simulink model "mpu6050_working_copy"  (R2017a)
settings: Solver=FixedStepDiscrete  StartTime=0.0  StopTime=inf  RelTol=1e-3
PostLoadFcn:
  | ChipSelect = 1;  % choose I2C comms
  | AddressAlt = 0;  % use default address
  | 
  | if AddressAlt == 1
  | % b1101001 (pin AD0 is logic high).
  | SlvAddr = uint8(bin2dec('1101001'));  % ADDR ALT = 1
  | else
  | % b1101000 (pin AD0 is logic low)
  | SlvAddr = uint8(bin2dec('1101000'));  % ADDR ALT = 0
  | end
  | SlvAddr = uint8(hex2dec('68'));
  | 
  | 
  | % 0x3B 59 ACCEL_XOUT[15:8]
  | % 0x3C 60 ACCEL_XOUT[7:0]
  | % 0x3D 61 ACCEL_YOUT[15:8]
  | % 0x3E 62 ACCEL_YOUT[7:0]
  | % 0x3F 63 ACCEL_ZOUT[15:8]
  | % 0x40 64 ACCEL_ZOUT[7:0]
  | 
  | AccelXRegAddr = uint8(hex2dec('3B'));
  | AccelYRegAddr = uint8(hex2dec('3D'));
  | AccelZRegAddr = uint8(hex2dec('3F'));
  | 
  | % 0x43 67 GYRO_XOUT[15:8]
  | % 0x44 68 GYRO_XOUT[7:0]
  | % 0x45 69 GYRO_YOUT[15:8]
  | % 0x46 70 GYRO_YOUT[7:0]
  | % 0x47 71 GYRO_ZOUT[15:8]
  | % 0x48 72 GYRO_ZOUT[7:0]
  | 
  | GyroXRegAddr = uint8(hex2dec('43'));
  | GyroYRegAddr = uint8(hex2dec('45'));
  | GyroZRegAddr = uint8(hex2dec('47'));
  | 
  | deviceAddr = fi(SlvAddr,0,7,0);
  | 
  | powerRegAddr = uint8(hex2dec('6B'));
  | powerRegData = bin2dec('10000001');
(part 2 of 2)

== stateflow chart mpu6050_working_copy/I2C_MPU6050_IP/MPU6050_Interface1 ==
  settings: executeAtInitialization=1
  state init
    %initstate
    Valid_Out = 0;
    selfInit = 1;
    slv_addr = SlvAddr;
    %TODO delete all
    tmp = 0;
    tmpConfig = 0;
    tmpReadGyro = 0;
    tmpReadAccel = 0;
    tmpValid = 0;
    tmpReadDevice = 0;
    tmpHere = 0;
  note: I2C Configuration for MPU6050
  note: 0x3B 59 ACCEL_XOUT[15:8]
      | 0x3C 60 ACCEL_XOUT[7:0]
      | 0x3D 61 ACCEL_YOUT[15:8]
      | 0x3E 62 ACCEL_YOUT[7:0]
      | 0x3F 63 ACCEL_ZOUT[15:8]
      | 0x40 64 ACCEL_ZOUT[7:0]
      |
      | 0x43 67 GYRO_XOUT[15:8]
      | 0x44 68 GYRO_XOUT[7:0]
      | 0x45 69 GYRO_YOUT[15:8]
      | 0x46 70 GYRO_YOUT[7:0]
      | 0x47 71 GYRO_ZOUT[15:8]
      | 0x48 72 GYRO_ZOUT[7:0]
      |
      | 0x6B 107 PWR_MGMT_1
      | 0x6C 108 PWR_MGMT_2
  state idle
    %idlestate
    enb 	= 0;
    rw 		= 0;
    mode 	= 0;
    cnt      = 0;
    reg_byte_mode = 0;
  state ReadDeviceData [group]
    note: DEVID is an example of
        | doing a 1-byte READ
    note: 0x75 117 - WHO_AM_I[6:1]
    state getDEVID
      entry:
      enb = 1;
      rw = 1;
      mode = 0;
      reg_addr =   uint8(117);
      tmpReadDevice = 1;
    state waitforNotBusy1
      enb=0;
    state readDEVID
      deviceId = uint8(data_in);
      tmpHere = 1;
    state waitforNotBusy6
      enb=0;
    state getRegData
      entry:
      enb = 1;
      rw = 1;
      mode = 0;
      reg_addr = userRegAddr;
    state waitforNotBusy5
      enb=0;
    state readUserRegData
      regdata = uint8(data_in);
    getDEVID -> waitforNotBusy1 : [busy==1]
    waitforNotBusy1 -> readDEVID [order 1] : [mstr_ack==1]
    waitforNotBusy1 -> waitforNotBusy6 [order 2] : [n_ack==1]
    readDEVID -> getRegData : [busy==0]
    waitforNotBusy6 -> (junction 2281) : [busy==0 || busy == 1]
    getRegData -> waitforNotBusy5 : [busy==1]
    waitforNotBusy5 -> readUserRegData [order 1] : [mstr_ack==1]
    waitforNotBusy5 -> (junction 2281) [order 2] : [n_ack==1]
  state Configuration [group]
    state setPwrMode
      enb = 1;
      rw = 0;
      mode = 0;
      reg_addr = powerRegAddr;
      data_out = powerRegData;
      tmpConfig = 1;
    state waitforNotBusy2
      enb=0;
    state setDataFormat [commented out]
      enb = 1;
      rw = 0;
      mode = 0;
      reg_addr = uint8(49); % 0x31
      data_out = uint8(0); % or 0x08
    state waitforNotBusy3 [commented out]
      enb=0;
    state setFIFOCfg [commented out]
      enb = 1;
      rw = 0;
      mode = 0;
      reg_addr = uint8(56); % 0x38
      data_out = uint8(8); % 0x08
    state waitforNotBusy4 [commented out]
      enb=0;
    state cfgDone
      selfInit = 0;
      tmp = 1;
    setPwrMode -> Configuration.waitforNotBusy2 : [busy==1]
    Configuration.waitforNotBusy2 -> (junction 2329) [order 2] : [busy==0]
    Configuration.waitforNotBusy2 -> (junction 2279) [order 1] : [n_ack==1]
    waitforNotBusy3 -> (junction 2279) [commented out] : [n_ack==1]
    waitforNotBusy4 -> (junction 2279) [commented out] : [n_ack==1]
    setDataFormat -> waitforNotBusy3 [commented out] : [busy==1]
    waitforNotBusy3 -> setFIFOCfg [commented out] : [busy==0]
    (junction 2329) -> Configuration.cfgDone
    setFIFOCfg -> waitforNotBusy4 [commented out] : [busy==1]
  state cfgDone
    selfInit = 0;
    tmp = 1;
  state check_cfg
    en: enb = 0;
    cnt = 0;
    du: cnt = cnt + 1;
    tmpCheckCng = 1
  state ReadAccelData [group]
    state read_accelX_registers0
      entry:
      enb = 1;
      rw = 1;
      mode = 1;
      reg_addr =  AccelXRegAddr;
      Valid_Out = 0;
      tmpReadAccel = 1;
    state waitforNotBusy2
      enb=0;
    state accelX_LSB
      tempVal = data_in;
    state toggle
    state accelX_MSB
      AccelX =  convert_int16(tempVal, data_in);
    state toggle3
    state accelY_LSB
      tempVal = data_in;
    state toggle1
    state accelY_MSB
      AccelY = convert_int16(tempVal,data_in);
    state toggle4
    state accelZ_LSB
      tempVal = data_in;
    state toggle2
      mode = 0;
    state accelZ_MSB
      AccelZ =  convert_int16(tempVal, data_in);
    read_accelX_registers0 -> ReadAccelData.waitforNotBusy2 : [busy==1]
    ReadAccelData.waitforNotBusy2 -> accelX_LSB [order 1] : [mstr_ack==1]
    accelX_LSB -> ReadAccelData.toggle : [mstr_ack==0]
    ReadAccelData.toggle -> accelX_MSB : [mstr_ack==1]
    accelX_MSB -> ReadAccelData.toggle3 [order 2] : [mstr_ack==0]
    accelX_MSB -> (junction 2286) [order 1] : [n_ack==1]
    ReadAccelData.toggle3 -> accelY_LSB : [mstr_ack==1]
    accelY_LSB -> ReadAccelData.toggle1 : [mstr_ack==0]
    ReadAccelData.toggle1 -> accelY_MSB : [mstr_ack==1]
    accelY_MSB -> (junction 2286) [order 1] : [n_ack==1]
    accelZ_MSB -> (junction 2286) [order 1] : [n_ack==1]
    accelY_MSB -> ReadAccelData.toggle4 [order 2] : [mstr_ack==0]
    ReadAccelData.toggle4 -> accelZ_LSB : [mstr_ack==1]
    accelZ_LSB -> ReadAccelData.toggle2 : [mstr_ack==0]
    ReadAccelData.toggle2 -> accelZ_MSB : [mstr_ack==1]
  state Valid
    en: enb = 0;
    cnt = 0;
    Valid_Out = 1;
    du: cnt = cnt + 1;
    tmpValid = 1;
  state ReadGyroData [group]
    state read_gyroX_registers0
      entry:
      enb = 1;
      rw = 1;
      mode = 1;
      reg_addr =  GyroXRegAddr;
      Valid_Out = 0;
      tmpReadGyro = 1;
    state waitforNotBusy2
      enb=0;
    state gyroX_LSB
      tempVal = data_in;
    state toggle
    state gyroX_MSB
      GyroX =  convert_int16(tempVal, data_in);
    state toggle3
    state gyroY_LSB
      tempVal = data_in;
    state toggle1
    state gyroY_MSB
      GyroY = convert_int16(tempVal, data_in);
    state toggle4
    state gyroZ_LSB
      tempVal = data_in;
    state toggle2
      mode = 0;
    state gyroZ_MSB
      GyroZ =  convert_int16(tempVal, data_in);
    read_gyroX_registers0 -> ReadGyroData.waitforNotBusy2 : [busy==1]
    ReadGyroData.waitforNotBusy2 -> gyroX_LSB : [mstr_ack==1]
    gyroX_LSB -> ReadGyroData.toggle : [mstr_ack==0]
    ReadGyroData.toggle -> gyroX_MSB : [mstr_ack==1]
    gyroX_MSB -> ReadGyroData.toggle3 [order 2] : [mstr_ack==0]
    gyroX_MSB -> (junction 2301) [order 1] : [n_ack==1]
    ReadGyroData.toggle3 -> gyroY_LSB : [mstr_ack==1]
    gyroY_LSB -> ReadGyroData.toggle1 : [mstr_ack==0]
    ReadGyroData.toggle1 -> gyroY_MSB : [mstr_ack==1]
    gyroY_MSB -> (junction 2301) [order 1] : [n_ack==1]
    gyroZ_MSB -> (junction 2301) [order 1] : [n_ack==1]
    gyroY_MSB -> ReadGyroData.toggle4 [order 2] : [mstr_ack==0]
    ReadGyroData.toggle4 -> gyroZ_LSB : [mstr_ack==1]
    gyroZ_LSB -> ReadGyroData.toggle2 : [mstr_ack==0]
    ReadGyroData.toggle2 -> gyroZ_MSB : [mstr_ack==1]
  (default) -> init
  init -> idle
  check_cfg -> idle : [cnt >=5]
  idle -> setPwrMode [order 1] : [busy==0 & (configDevice==1 | selfInit == 1)]
  idle -> getDEVID [order 2] : [busy==0]
  readUserRegData -> read_accelX_registers0 : [busy==0]
  (junction 2281) -> check_cfg
  (junction 2286) -> check_cfg
  (junction 2279) -> check_cfg
  ReadAccelData.waitforNotBusy2 -> check_cfg [order 2] : [n_ack==1]
  Valid -> check_cfg : [cnt >= 5]
  Configuration.cfgDone -> read_accelX_registers0
  accelZ_MSB -> read_gyroX_registers0 [order 2] : [busy==0]
  gyroZ_MSB -> Valid [order 2]
  data: msb function_input uint8; lsb function_input uint8; val function_output int16; enb output boolean size=1; rw output boolean size=1; mode output boolean size=1; slv_addr output uint8; reg_addr output uint8; reg_byte_mode output boolean size=1; data_out output uint8; busy input; n_ack input; byte_mode input boolean size=1; reg_mode input boolean size=1; cnt local uint32; data_in input uint8 size=1; mstr_ack input; AccelX output int16; AccelY output int16; AccelZ output int16; SlvAddr parameter uint8; AccelXRegAddr parameter uint8; AccelYRegAddr parameter uint8; AccelZRegAddr parameter uint8; Valid_Out output boolean; tempVal local uint8; deviceId output uint8; powerRegData parameter uint8; regdata output uint8; userRegAddr input uint8; powerRegAddr parameter uint8; configDevice input boolean; selfInit local boolean; GyroXRegAddr parameter uint8; GyroX output int16; GyroY output int16; GyroZ output int16; tmp output boolean; tmpConfig output boolean; tmpCheckCng output boolean; tmpReadGyro output boolean; tmpReadAccel output boolean; tmpValid output boolean; tmpReadDevice output boolean; tmpHere output boolean
  function val = convert_int16(msb, lsb):
    | function val = convert_int16(msb, lsb)
    | 
    | val = int16(bitor(bitshift(int16(msb),8), int16(lsb)));

== stateflow chart mpu6050_working_copy/I2C_MPU6050_IP/MPU6050_Interface2 ==
  settings: executeAtInitialization=1
  state init
    %initstate
    Valid_Out = 0;
    selfInit = 1;
    slv_addr = SlvAddr;
    %TODO delete all
    tmp = 0;
    tmpConfig = 0;
    tmpReadGyro = 0;
    tmpReadAccel = 0;
    tmpValid = 0;
    tmpReadDevice = 0;
    tmpHere = 0;
  state idle1 [commented out]
    %idlestate
    enb 	= 0;
    rw 		= 0;
    mode 	= 0;
    cnt      = 0;
    reg_byte_mode = 0;
  state WriteByteExample [group] [commented out]
    state exPowerMOde [commented out]
      enb = 1;
      rw = 0;
      mode = 0;
      reg_addr = hex2dec('6B');
      data_out = hex2dec('80');
    state waitforNotBusy2 [commented out]
      enb=0;
    state waitforNotBusy3 [commented out]
      enb=0;
    exPowerMOde -> WriteByteExample.waitforNotBusy2 [commented out] : [busy==1]
    WriteByteExample.waitforNotBusy2 -> WriteByteExample.waitforNotBusy3 [commented out] : [busy==0]
  note: I2C Configuration for MPU6050
  note: 0x3B 59 ACCEL_XOUT[15:8]
      | 0x3C 60 ACCEL_XOUT[7:0]
      | 0x3D 61 ACCEL_YOUT[15:8]
      | 0x3E 62 ACCEL_YOUT[7:0]
      | 0x3F 63 ACCEL_ZOUT[15:8]
      | 0x40 64 ACCEL_ZOUT[7:0]
      |
      | 0x43 67 GYRO_XOUT[15:8]
      | 0x44 68 GYRO_XOUT[7:0]
      | 0x45 69 GYRO_YOUT[15:8]
      | 0x46 70 GYRO_YOUT[7:0]
      | 0x47 71 GYRO_ZOUT[15:8]
      | 0x48 72 GYRO_ZOUT[7:0]
      |
      | 0x6B 107 PWR_MGMT_1
      | 0x6C 108 PWR_MGMT_2
  state idle
    %idlestate
    enb 	= 0;
    rw 		= 0;
    mode 	= 0;
    cnt      = 0;
    reg_byte_mode = 0;
  state ReadDeviceData [group]
    note: DEVID is an example of
        | doing a 1-byte READ
    note: 0x75 117 - WHO_AM_I[6:1]
    state getDEVID
      entry:
      enb = 1;
      rw = 1;
      mode = 0;
      reg_addr =   uint8(117);
      tmpReadDevice = 1;
    state waitforNotBusy1
      enb=0;
    state readDEVID
      deviceId = uint8(data_in);
      tmpHere = 1;
    state waitforNotBusy6
      enb=0;
    state getRegData
      entry:
      enb = 1;
      rw = 1;
      mode = 0;
      reg_addr = userRegAddr;
    state waitforNotBusy5
      enb=0;
    state readUserRegData
      regdata = uint8(data_in);
    getDEVID -> waitforNotBusy1 : [busy==1]
    waitforNotBusy1 -> readDEVID [order 1] : [mstr_ack==1]
    waitforNotBusy1 -> ReadDeviceData.waitforNotBusy6 [order 2] : [n_ack==1]
    readDEVID -> getRegData : [busy==0]
    ReadDeviceData.waitforNotBusy6 -> (junction 2281) : [busy==0 || busy == 1]
    getRegData -> ReadDeviceData.waitforNotBusy5 : [busy==1]
    ReadDeviceData.waitforNotBusy5 -> readUserRegData [order 1] : [mstr_ack==1]
    ReadDeviceData.waitforNotBusy5 -> (junction 2281) [order 2] : [n_ack==1]
  state Configuration [group]
    state setPwrMode
      enb = 1;
      rw = 0;
      mode = 0;
      reg_addr = powerRegAddr;
      data_out = powerRegData;
      tmpConfig = 1;
    state waitforNotBusy2
      enb=0;
    state setDataFormat [commented out]
      enb = 1;
      rw = 0;
      mode = 0;
      reg_addr = uint8(49); % 0x31
      data_out = uint8(0); % or 0x08
    state waitforNotBusy3 [commented out]
      enb=0;
    state setFIFOCfg [commented out]
      enb = 1;
      rw = 0;
      mode = 0;
      reg_addr = uint8(56); % 0x38
      data_out = uint8(8); % 0x08
    state waitforNotBusy4 [commented out]
      enb=0;
    state cfgDone
      selfInit = 0;
      tmp = 1;
    setPwrMode -> Configuration.waitforNotBusy2 : [busy==1]
    Configuration.waitforNotBusy2 -> (junction 2329) [order 2] : [busy==0]
    Configuration.waitforNotBusy2 -> (junction 2279) [order 1] : [n_ack==1]
    Configuration.waitforNotBusy3 -> (junction 2279) [commented out] : [n_ack==1]
    Configuration.waitforNotBusy4 -> (junction 2279) [commented out] : [n_ack==1]
    setDataFormat -> Configuration.waitforNotBusy3 [commented out] : [busy==1]
    Configuration.waitforNotBusy3 -> setFIFOCfg [commented out] : [busy==0]
    (junction 2329) -> cfgDone
    setFIFOCfg -> Configuration.waitforNotBusy4 [commented out] : [busy==1]
  state check_cfg
    en: enb = 0;
    cnt = 0;
    du: cnt = cnt + 1;
    tmpCheckCng = 1
  state ReadAccelData [group]
    state read_accelX_registers0
      entry:
      enb = 1;
      rw = 1;
      mode = 1;
      reg_addr =  AccelXRegAddr;
      Valid_Out = 0;
      tmpReadAccel = 1;
    state waitforNotBusy2
      enb=0;
    state accelX_LSB
      tempVal = data_in;
    state toggle
    state accelX_MSB
      AccelX =  convert_int16(tempVal, data_in);
    state toggle3
    state accelY_LSB
      tempVal = data_in;
    state toggle1
    state accelY_MSB
      AccelY = convert_int16(tempVal,data_in);
    state toggle4
    state accelZ_LSB
      tempVal = data_in;
    state toggle2
      mode = 0;
    state accelZ_MSB
      AccelZ =  convert_int16(tempVal, data_in);
    read_accelX_registers0 -> ReadAccelData.waitforNotBusy2 : [busy==1]
    ReadAccelData.waitforNotBusy2 -> accelX_LSB [order 1] : [mstr_ack==1]
    accelX_LSB -> ReadAccelData.toggle : [mstr_ack==0]
    ReadAccelData.toggle -> accelX_MSB : [mstr_ack==1]
    accelX_MSB -> ReadAccelData.toggle3 [order 2] : [mstr_ack==0]
    accelX_MSB -> (junction 2286) [order 1] : [n_ack==1]
    ReadAccelData.toggle3 -> accelY_LSB : [mstr_ack==1]
    accelY_LSB -> ReadAccelData.toggle1 : [mstr_ack==0]
    ReadAccelData.toggle1 -> accelY_MSB : [mstr_ack==1]
    accelY_MSB -> (junction 2286) [order 1] : [n_ack==1]
    accelZ_MSB -> (junction 2286) [order 1] : [n_ack==1]
    accelY_MSB -> ReadAccelData.toggle4 [order 2] : [mstr_ack==0]
    ReadAccelData.toggle4 -> accelZ_LSB : [mstr_ack==1]
    accelZ_LSB -> ReadAccelData.toggle2 : [mstr_ack==0]
    ReadAccelData.toggle2 -> accelZ_MSB : [mstr_ack==1]
  state WriteByteExample [group] [commented out]
    state waitforNotBusy4 [commented out]
      enb=0;
    state resetPowerMode [commented out]
      enb = 1;
      rw = 0;
      mode = 0;
      reg_addr = 107; %0x6B
      data_out = 128; %0x80
    state setClockSource1 [commented out]
      enb = 1;
      rw = 0;
      mode = 0;
      reg_addr = 107; %0x6B
      data_out = 1; %0x01
    state waitforNotBusy5 [commented out]
      enb=0;
    state setClockSource2Maybe [commented out]
      enb = 1;
      rw = 0;
      mode = 0;
      reg_addr = 108; %0x6C
      data_out = 0; %0x00
    state waitforNotBusy6 [commented out]
      enb=0;
    state clearSleepEnableSensors [commented out]
      enb = 1;
      rw = 0;
      mode = 0;
      reg_addr = 107; %0x6B
      data_out = 0; %0x0
    state waitforNotBusy6B [commented out]
      enb=0;
    state configGyroAndAccel1 [commented out]
      enb = 1;
      rw = 0;
      mode = 0;
      reg_addr = 107; %0x6B
      data_out = 1; %0x01
    state waitforNotBusy7 [commented out]
      enb=0;
    state configGyroAndAccel [commented out]
      enb = 1;
      rw = 0;
      mode = 0;
      reg_addr = 26; %0x1A
      data_out = 3; %0x03
    state waitforNotBusy8 [commented out]
      enb=0;
    state setSampleRate [commented out]
      %200hz
      enb = 1;
      rw = 0;
      mode = 0;
      reg_addr = 25; %0x19
      data_out = 4; %0x04
    state waitforNotBusy9 [commented out]
      enb=0;
    state setupInterrupts [commented out]
      enb = 1;
      rw = 0;
      mode = 0;
      reg_addr = 55; %0x37
      data_out = 2; %0x02
    state waitforNotBusy10 [commented out]
      enb=0;
    state enableInterrupts [commented out]
      enb = 1;
      rw = 0;
      mode = 0;
      reg_addr = 56; %0x38
      data_out = 1; %0x01
    WriteByteExample.waitforNotBusy4 -> WriteByteExample.setClockSource1 [commented out] : [busy==0]
    WriteByteExample.resetPowerMode -> WriteByteExample.waitforNotBusy4 [commented out] : [busy==1]
    WriteByteExample.setClockSource1 -> WriteByteExample.waitforNotBusy5 [commented out] : [busy==1]
    WriteByteExample.waitforNotBusy5 -> WriteByteExample.setClockSource2Maybe [commented out] : [busy==0]
    WriteByteExample.waitforNotBusy6 -> WriteByteExample.clearSleepEnableSensors [commented out] : [busy==0]
    WriteByteExample.setClockSource2Maybe -> WriteByteExample.waitforNotBusy6 [commented out] : [busy==1]
    WriteByteExample.clearSleepEnableSensors -> WriteByteExample.waitforNotBusy6B [commented out] : [busy==1]
    WriteByteExample.waitforNotBusy6B -> WriteByteExample.configGyroAndAccel1 [commented out] : [busy==0]
    WriteByteExample.waitforNotBusy7 -> configGyroAndAccel [commented out] : [busy==0]
    WriteByteExample.configGyroAndAccel1 -> WriteByteExample.waitforNotBusy7 [commented out] : [busy==1]
    waitforNotBusy8 -> setSampleRate [commented out] : [busy==0]
    configGyroAndAccel -> waitforNotBusy8 [commented out] : [busy==1]
    setSampleRate -> waitforNotBusy9 [commented out] : [busy==1]
    waitforNotBusy9 -> setupInterrupts [commented out] : [busy==0]
    waitforNotBusy10 -> enableInterrupts [commented out] : [busy==0]
    setupInterrupts -> waitforNotBusy10 [commented out] : [busy==1]
  state WriteByteExample [group]
    state waitforNotBusy4
      enb=0;
    state resetPowerMode
      enb = 1;
      rw = 0;
      mode = 0;
      reg_addr = 107; %0x6B
      data_out = 128; %0x80
    state setClockSource1
      enb = 1;
      rw = 0;
      mode = 0;
      reg_addr = 107; %0x6B
      data_out = 1; %0x01
    state waitforNotBusy5
      enb=0;
    state setClockSource2Maybe
      enb = 1;
      rw = 0;
      mode = 0;
      reg_addr = 108; %0x6C
      data_out = 0; %0x00
    state waitforNotBusy6
      enb=0;
    state clearSleepEnableSensors
      enb = 1;
      rw = 0;
      mode = 0;
      reg_addr = 27; %0x6B
      data_out = 0; %0x0
    state waitforNotBusy6B
      enb=0;
    state configGyroAndAccel1
      enb = 1;
      rw = 0;
      mode = 0;
      reg_addr = 28; %0x6B
      data_out = 0; %0x01
    state waitforNotBusy7
      enb=0;
    WriteByteExample.waitforNotBusy4 -> WriteByteExample.setClockSource1 : [busy==0]
    WriteByteExample.resetPowerMode -> WriteByteExample.waitforNotBusy4 : [busy==1]
    WriteByteExample.setClockSource1 -> WriteByteExample.waitforNotBusy5 : [busy==1]
    WriteByteExample.waitforNotBusy5 -> WriteByteExample.setClockSource2Maybe : [busy==0]
    WriteByteExample.waitforNotBusy6 -> WriteByteExample.clearSleepEnableSensors : [busy==0]
    WriteByteExample.setClockSource2Maybe -> WriteByteExample.waitforNotBusy6 : [busy==1]
    WriteByteExample.clearSleepEnableSensors -> WriteByteExample.waitforNotBusy6B : [busy==1]
    WriteByteExample.waitforNotBusy6B -> WriteByteExample.configGyroAndAccel1 : [busy==0]
    WriteByteExample.configGyroAndAccel1 -> WriteByteExample.waitforNotBusy7 : [busy==1]
  state Valid
    en: enb = 0;
    cnt = 0;
    Valid_Out = 1;
    du: cnt = cnt + 1;
    tmpValid = 1;
  state ReadGyroData [group]
    state read_gyroX_registers0
      entry:
      enb = 1;
      rw = 1;
      mode = 1;
      reg_addr =  GyroXRegAddr;
      Valid_Out = 0;
      tmpReadGyro = 1;
    state waitforNotBusy2
      enb=0;
    state gyroX_LSB
      tempVal = data_in;
    state toggle
    state gyroX_MSB
      GyroX =  convert_int16(tempVal, data_in);
    state toggle3
    state gyroY_LSB
      tempVal = data_in;
    state toggle1
    state gyroY_MSB
      GyroY = convert_int16(tempVal, data_in);
    state toggle4
    state gyroZ_LSB
      tempVal = data_in;
    state toggle2
      mode = 0;
    state gyroZ_MSB
      GyroZ =  convert_int16(tempVal, data_in);
    read_gyroX_registers0 -> ReadGyroData.waitforNotBusy2 : [busy==1]
    ReadGyroData.waitforNotBusy2 -> gyroX_LSB : [mstr_ack==1]
    gyroX_LSB -> ReadGyroData.toggle : [mstr_ack==0]
    ReadGyroData.toggle -> gyroX_MSB : [mstr_ack==1]
    gyroX_MSB -> ReadGyroData.toggle3 [order 2] : [mstr_ack==0]
    gyroX_MSB -> (junction 2301) [order 1] : [n_ack==1]
    ReadGyroData.toggle3 -> gyroY_LSB : [mstr_ack==1]
    gyroY_LSB -> ReadGyroData.toggle1 : [mstr_ack==0]
    ReadGyroData.toggle1 -> gyroY_MSB : [mstr_ack==1]
    gyroY_MSB -> (junction 2301) [order 1] : [n_ack==1]
    gyroZ_MSB -> (junction 2301) [order 1] : [n_ack==1]
    gyroY_MSB -> ReadGyroData.toggle4 [order 2] : [mstr_ack==0]
    ReadGyroData.toggle4 -> gyroZ_LSB : [mstr_ack==1]
    gyroZ_LSB -> ReadGyroData.toggle2 : [mstr_ack==0]
    ReadGyroData.toggle2 -> gyroZ_MSB : [mstr_ack==1]
  (default) -> init
  idle1 -> exPowerMOde [commented out]
  init -> idle
  check_cfg -> idle : [cnt >=5]
  idle -> setPwrMode [order 1] : [busy==0 && (configDevice==1 || selfInit == 1)]
  idle -> getDEVID [order 2] : [busy==0]
  readUserRegData -> read_accelX_registers0 : [busy==0]
  (junction 2281) -> check_cfg
  (junction 2286) -> check_cfg
  (junction 2279) -> check_cfg
  ReadAccelData.waitforNotBusy2 -> check_cfg [order 2] : [n_ack==1]
  Valid -> check_cfg : [cnt >= 5]
  cfgDone -> read_accelX_registers0 [commented out]
  enableInterrupts -> ? [commented out]
  WriteByteExample.waitforNotBusy7 -> read_accelX_registers0
  (default) -> WriteByteExample.resetPowerMode [commented out]
  cfgDone -> WriteByteExample.resetPowerMode
  accelZ_MSB -> read_gyroX_registers0 [order 2] : [busy==0]
  gyroZ_MSB -> Valid [order 2]
  data: msb function_input uint8; lsb function_input uint8; val function_output int16; enb output boolean size=1; rw output boolean size=1; mode output boolean size=1; slv_addr output uint8; reg_addr output uint8; reg_byte_mode output boolean size=1; data_out output uint8; busy input; n_ack input; byte_mode input boolean size=1; reg_mode input boolean size=1; cnt local uint32; data_in input uint8 size=1; mstr_ack input; AccelX output int16; AccelY output int16; AccelZ output int16; SlvAddr parameter uint8; AccelXRegAddr parameter uint8; AccelYRegAddr parameter uint8; AccelZRegAddr parameter uint8; Valid_Out output boolean; tempVal local uint8; deviceId output uint8; powerRegData parameter uint8; regdata output uint8; userRegAddr input uint8; powerRegAddr parameter uint8; configDevice input boolean; selfInit local boolean; GyroXRegAddr parameter uint8; GyroX output int16; GyroY output int16; GyroZ output int16; tmp output boolean; tmpConfig output boolean; tmpCheckCng output boolean; tmpReadGyro output boolean; tmpReadAccel output boolean; tmpValid output boolean; tmpReadDevice output boolean; tmpHere output boolean
  function val = convert_int16(msb, lsb):
    | function val = convert_int16(msb, lsb)
    | 
    | val = int16(bitor(bitshift(int16(msb),8), int16(lsb)));

== matlab function mpu6050_working_copy/AngleConverterX/MATLAB Function1 ==
  data: inAngle input; angle output; isDeviceSetup input
function angle = fcn(inAngle, isDeviceSetup)
    if isDeviceSetup == true
        angle = inAngle;
    else
        angle = 0;
    end
